simulink model "ex9"  (Simulink 6.3)
settings: Solver=VariableStepDiscrete  StartTime=0.0  StopTime=1  RelTol=1e-3
values from neighbouring files (symbols this model uses):
  BER = ber(ii)    [ex7sim.m]    (also in ex9sim.m)
undefined symbols (not defined in the file or in its folder): CRC
libraries: commcrc2 x2, commrandsrc2 x1, commchan3 x1, dspmathops x1, commsink2 x1, dspsnks4 x1
settings Model: LastModifiedBy=lxy  StrictBusMsg=None
settings OptimizationCC: InlineInvariantSignals=on

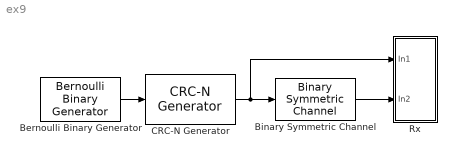
== system ex9 ==
  Bernoulli Binary Generator : commrandsrc2/Bernoulli Binary Generator  P=0.5  seed=61  Ts=1/6400000  frameBased=on  sampPerFrame=64  orient=off  outDataType=double
  Binary Symmetric Channel : commchan3/Binary Symmetric Channel  P=BER  s=71  E=off  outDtype=double
  CRC-N Generator : commcrc2/CRC-N Generator  crcMethod=CRC-16  iniStates=[0]  numChecksums=1
  Rx : Subsystem
  wires:
  Bernoulli Binary Generator/1 -> CRC-N Generator/1
  Binary Symmetric Channel/1 -> Rx/2(In2)
  CRC-N Generator/1 -> Binary Symmetric Channel/1, Rx/1(In1)

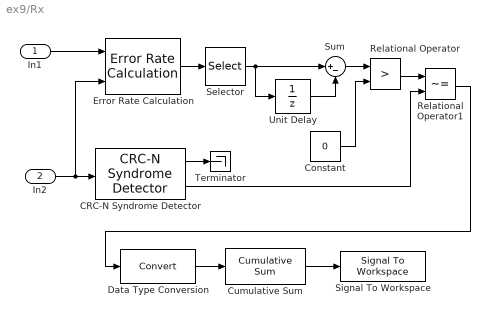
== system ex9/Rx ==
  In1 : Inport
  In2 : Inport  Port=2
  CRC-N Syndrome Detector : commcrc2/CRC-N Syndrome Detector  crcMethod=CRC-16  iniStates=[0]  numChecksums=1
  Constant : Constant  Value=0
  Cumulative Sum : dspmathops/Cumulative Sum  DialogController=dspDDGCreate  DialogControllerArgs=DataTag0  dim=Channels (running sum)  reset_popup=None  roundingMode=Floor  overflowMode=off
  Data Type Conversion : DataTypeConversion
  Error Rate Calculation : commsink2/Error Rate Calculation  N=0  st_delay=0  cp_mode=Entire frame  subframe=[]  PMode=Port  WsName=BER1  RsMode2=off  stop=off  numErr=100  maxBits=1e6
  Relational Operator : RelationalOperator  Operator=>  LogicOutDataTypeMode=Boolean
  Relational Operator1 : RelationalOperator  Operator=~=  LogicOutDataTypeMode=Boolean
  Selector : Selector  Elements=[2]  InputPortWidth=3
  Signal To Workspace : dspsnks4/Signal To Workspace  VariableName=MissedFrame  FrameMode=Concatenate frames (2-D array)
      settings: FixptAsFi=off
  Sum : Sum  Inputs=|+-
  Terminator : Terminator
  Unit Delay : UnitDelay  SampleTime=-1
  wires:
  In2/1 -> CRC-N Syndrome Detector/1, Error Rate Calculation/2
  CRC-N Syndrome Detector/1 -> Terminator/1
  CRC-N Syndrome Detector/2 -> Relational Operator1/2
  Error Rate Calculation/1 -> Selector/1
  Selector/1 -> Unit Delay/1, Sum/1
  Unit Delay/1 -> Sum/2
  Constant/1 -> Relational Operator/2
  Relational Operator/1 -> Relational Operator1/1
  In1/1 -> Error Rate Calculation/1
  Sum/1 -> Relational Operator/1
  Data Type Conversion/1 -> Cumulative Sum/1
  Cumulative Sum/1 -> Signal To Workspace/1
  Relational Operator1/1 -> Data Type Conversion/1
